simulink library "motor_interface_lib"  (R2022b)
settings: Solver=VariableStepAuto  StartTime=0.0  StopTime=10.0  RelTol=1e-3
undefined symbols (not defined in the file): MI_STATUSES
settings Model: Creator=dr_pa  LastModifiedBy=LinF

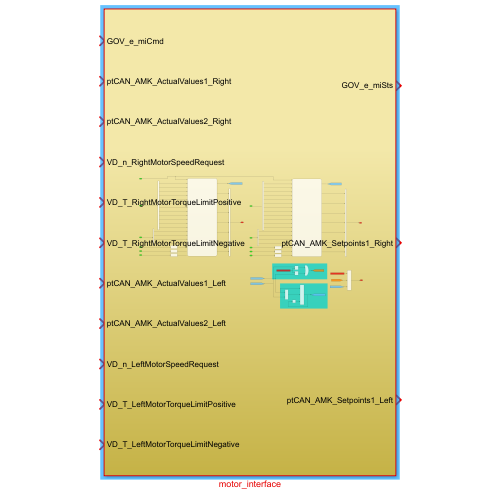
[thumbnail: Simulink's stored preview of the top-level diagram]
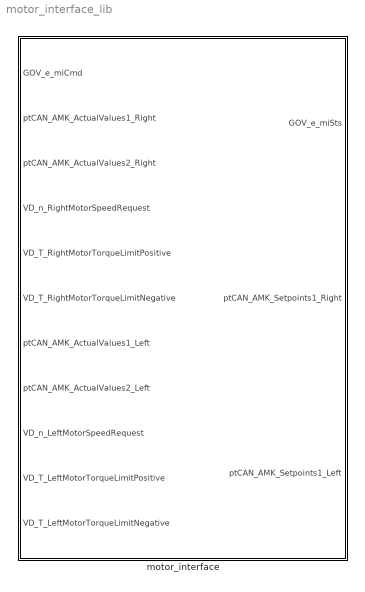
== system motor_interface_lib ==
  motor_interface : Subsystem

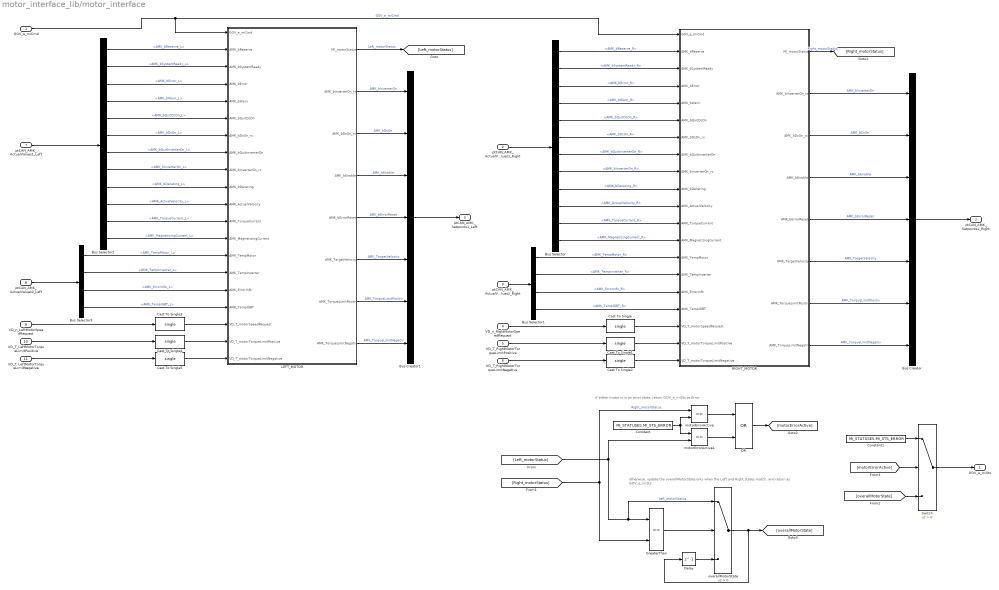
== system motor_interface_lib/motor_interface ==
  note: otherwise, update the overallMotorState only when the Left and Right states match, and return as GOV_e_miSts
  note: if either motor is in an error state, return GOV_e_miSts as Error
  GOV_e_miCmd : Inport
  ptCAN_AMK_ActualValues1_Right : Inport  Port=2
  ptCAN_AMK_ActualValues2_Right : Inport  Port=3
  VD_n_RightMotorSpeedRequest : Inport  Port=4
  VD_T_RightMotorTorqueLimitPositive : Inport  Port=5
  VD_T_RightMotorTorqueLimitNegative : Inport  Port=6
  ptCAN_AMK_ActualValues1_Left : Inport  Port=7
  ptCAN_AMK_ActualValues2_Left : Inport  Port=8
  VD_n_LeftMotorSpeedRequest : Inport  Port=9
  VD_T_LeftMotorTorqueLimitPositive : Inport  Port=10
  VD_T_LeftMotorTorqueLimitNegative : Inport  Port=11
  Bus Creator : BusCreator  Inputs=7
  Bus Creator1 : BusCreator  Inputs=7
  Bus Selector : BusSelector  OutputSignals=AMK_bReserve_R,AMK_bSystemReady_R,AMK_bError_R,AMK_bWarn_R,AMK_bQuitDcOn_R,AMK_bDcOn_R,AMK_bQuitInverterOn_R,AMK_bInverterOn_R,AMK_bDerating_R,AMK_ActualVelocity_R,AMK_TorqueCurrent_R,AMK_MagnetizingCurrent_R
  Bus Selector1 : BusSelector  OutputSignals=AMK_TempMotor_R,AMK_TempInverter_R,AMK_ErrorInfo_R,AMK_TempIGBT_R
  Bus Selector2 : BusSelector  OutputSignals=AMK_bReserve_L,AMK_bSystemReady_L,AMK_bError_L,AMK_bWarn_L,AMK_bQuitDcOn_L,AMK_bDcOn_L,AMK_bQuitInverterOn_L,AMK_bInverterOn_L,AMK_bDerating_L,AMK_ActualVelocity_L,AMK_TorqueCurrent_L,AMK_MagnetizingCurrent_L
  Bus Selector3 : BusSelector  OutputSignals=AMK_TempMotor_L,AMK_TempInverter_L,AMK_ErrorInfo_L,AMK_TempIGBT_L
  Cast To Single{,1..5} (6 alike) : DataTypeConversion  OutDataTypeStr=single  SaturateOnIntegerOverflow=off  RndMeth=Floor
  Constant : Constant  Value=MI_STATUSES.MI_STS_ERROR  OutDataTypeStr=Enum: MI_STATUSES
  Constant1 : Constant  Value=MI_STATUSES.MI_STS_ERROR  OutDataTypeStr=Enum: MI_STATUSES
  Delay : Delay  DelayLength=1  InitialCondition=MI_STATUSES.OFF
  GreaterThan : RelationalOperator  Operator===  OutDataTypeStr=boolean  RndMeth=Simplest  InputSameDT=off
  LEFT_MOTOR : Stateflow chart  TreatAsAtomicUnit=on
  OR : Logic  Operator=OR  IconShape=distinctive  AllPortsSameDT=off  OutDataTypeStr=boolean
  RIGHT_MOTOR : Stateflow chart  TreatAsAtomicUnit=on
  Switch : Switch  Criteria=u2 > Threshold  SaturateOnIntegerOverflow=off  InputSameDT=off
  motorErrorActive : RelationalOperator  Operator===  OutDataTypeStr=boolean  RndMeth=Simplest  InputSameDT=off
  motorErrorActive1 : RelationalOperator  Operator===  OutDataTypeStr=boolean  RndMeth=Simplest  InputSameDT=off
  overallMotorState : Switch  Criteria=u2 > Threshold  SaturateOnIntegerOverflow=off  InputSameDT=off
  GOV_e_miSts : Outport
  ptCAN_AMK_Setpoints1_Right : Outport  Port=2
  ptCAN_AMK_Setpoints1_Left : Outport  Port=3
  wires:
  Cast To Single5/1 -> LEFT_MOTOR/20(VD_T_motorTorqueLimitNegative)
  Cast To Single4/1 -> LEFT_MOTOR/19(VD_T_motorTorqueLimitPositive)
  Cast To Single3/1 -> LEFT_MOTOR/18(VD_T_motorSpeedRequest)
  Cast To Single2/1 -> RIGHT_MOTOR/20(VD_T_motorTorqueLimitNegative)
  Cast To Single1/1 -> RIGHT_MOTOR/19(VD_T_motorTorqueLimitPositive)
  Cast To Single/1 -> RIGHT_MOTOR/18(VD_T_motorSpeedRequest)
  GOV_e_miCmd/1 -> LEFT_MOTOR/1(GOV_e_miCmd), RIGHT_MOTOR/1(GOV_e_miCmd)  "GOV_e_miCmd"
  ptCAN_AMK_ActualValues1_Right/1 -> Bus Selector/1
  Bus Selector/2 -> RIGHT_MOTOR/3(AMK_bSystemReady)  "<AMK_bSystemReady_R>"
  Bus Selector/3 -> RIGHT_MOTOR/4(AMK_bError)  "<AMK_bError_R>"
  Bus Selector/4 -> RIGHT_MOTOR/5(AMK_bWarn)  "<AMK_bWarn_R>"
  Bus Selector/5 -> RIGHT_MOTOR/6(AMK_bQuitDcOn)  "<AMK_bQuitDcOn_R>"
  Bus Selector/6 -> RIGHT_MOTOR/7(AMK_bDcOn_rx)  "<AMK_bDcOn_R>"
  Bus Selector/7 -> RIGHT_MOTOR/8(AMK_bQuitInverterOn)  "<AMK_bQuitInverterOn_R>"
  Bus Selector/8 -> RIGHT_MOTOR/9(AMK_bInverterOn_rx)  "<AMK_bInverterOn_R>"
  Bus Selector/9 -> RIGHT_MOTOR/10(AMK_bDerating)  "<AMK_bDerating_R>"
  Bus Selector/10 -> RIGHT_MOTOR/11(AMK_ActualVelocity)  "<AMK_ActualVelocity_R>"
  Bus Selector/11 -> RIGHT_MOTOR/12(AMK_TorqueCurrent)  "<AMK_TorqueCurrent_R>"
  Bus Selector/12 -> RIGHT_MOTOR/13(AMK_MagnetizingCurrent)  "<AMK_MagnetizingCurrent_R>"
  Bus Selector/1 -> RIGHT_MOTOR/2(AMK_bReserve)  "<AMK_bReserve_R>"
  ptCAN_AMK_ActualValues2_Right/1 -> Bus Selector1/1
  Bus Selector1/1 -> RIGHT_MOTOR/14(AMK_TempMotor)  "<AMK_TempMotor_R>"
  Bus Selector1/2 -> RIGHT_MOTOR/15(AMK_TempInverter)  "<AMK_TempInverter_R>"
  Bus Selector1/3 -> RIGHT_MOTOR/16(AMK_ErrorInfo)  "<AMK_ErrorInfo_R>"
  Bus Selector1/4 -> RIGHT_MOTOR/17(AMK_TempIGBT)  "<AMK_TempIGBT_R>"
  Bus Creator/1 -> ptCAN_AMK_Setpoints1_Right/1
  RIGHT_MOTOR/2(AMK_bInverterOn_tx) -> Bus Creator/1  "AMK_bInverterOn"
  RIGHT_MOTOR/4(AMK_bEnable) -> Bus Creator/3  "AMK_bEnable"
  RIGHT_MOTOR/6(AMK_TargetVelocity) -> Bus Creator/5  "AMK_TargetVelocity"
  RIGHT_MOTOR/3(AMK_bDcOn_tx) -> Bus Creator/2  "AMK_bDcOn"
  RIGHT_MOTOR/5(AMK_bErrorReset) -> Bus Creator/4  "AMK_bErrorReset"
  LEFT_MOTOR/1(MI_motorStatus) -> [Left_motorStatus]  "Left_motorStatus"
  RIGHT_MOTOR/1(MI_motorStatus) -> [Right_motorStatus]  "Right_motorStatus"
  [Left_motorStatus] -> motorErrorActive1/2, overallMotorState/1, GreaterThan/1  "Left_motorStatus"
  [Right_motorStatus] -> motorErrorActive/1, GreaterThan/2  "Right_motorStatus"
  Constant/1 -> motorErrorActive/2, motorErrorActive1/1
  Switch/1 -> GOV_e_miSts/1
  [motorErrorActive] -> Switch/2
  overallMotorState/1 -> Delay/1, [overallMotorState]
  Delay/1 -> overallMotorState/3
  GreaterThan/1 -> overallMotorState/2
  [overallMotorState] -> Switch/3
  OR/1 -> [motorErrorActive]
  motorErrorActive1/1 -> OR/2
  motorErrorActive/1 -> OR/1
  Constant1/1 -> Switch/1
  RIGHT_MOTOR/7(AMK_TorqueLimitPositiv) -> Bus Creator/6  "AMK_TorqueLimitPositiv"
  RIGHT_MOTOR/8(AMK_TorqueLimitNegativ) -> Bus Creator/7  "AMK_TorqueLimitNegativ"
  VD_T_RightMotorTorqueLimitPositive/1 -> Cast To Single1/1
  VD_T_RightMotorTorqueLimitNegative/1 -> Cast To Single2/1
  VD_n_RightMotorSpeedRequest/1 -> Cast To Single/1
  VD_n_LeftMotorSpeedRequest/1 -> Cast To Single3/1
  VD_T_LeftMotorTorqueLimitNegative/1 -> Cast To Single5/1
  VD_T_LeftMotorTorqueLimitPositive/1 -> Cast To Single4/1
  Bus Selector3/4 -> LEFT_MOTOR/17(AMK_TempIGBT)  "<AMK_TempIGBT_L>"
  Bus Selector3/3 -> LEFT_MOTOR/16(AMK_ErrorInfo)  "<AMK_ErrorInfo_L>"
  Bus Selector3/2 -> LEFT_MOTOR/15(AMK_TempInverter)  "<AMK_TempInverter_L>"
  Bus Selector3/1 -> LEFT_MOTOR/14(AMK_TempMotor)  "<AMK_TempMotor_L>"
  Bus Selector2/1 -> LEFT_MOTOR/2(AMK_bReserve)  "<AMK_bReserve_L>"
  Bus Selector2/12 -> LEFT_MOTOR/13(AMK_MagnetizingCurrent)  "<AMK_MagnetizingCurrent_L>"
  Bus Selector2/11 -> LEFT_MOTOR/12(AMK_TorqueCurrent)  "<AMK_TorqueCurrent_L>"
  Bus Selector2/10 -> LEFT_MOTOR/11(AMK_ActualVelocity)  "<AMK_ActualVelocity_L>"
  Bus Selector2/9 -> LEFT_MOTOR/10(AMK_bDerating)  "<AMK_bDerating_L>"
  Bus Selector2/8 -> LEFT_MOTOR/9(AMK_bInverterOn_rx)  "<AMK_bInverterOn_L>"
  Bus Selector2/7 -> LEFT_MOTOR/8(AMK_bQuitInverterOn)  "<AMK_bQuitInverterOn_L>"
  Bus Selector2/6 -> LEFT_MOTOR/7(AMK_bDcOn_rx)  "<AMK_bDcOn_L>"
  Bus Selector2/5 -> LEFT_MOTOR/6(AMK_bQuitDcOn)  "<AMK_bQuitDcOn_L>"
  Bus Selector2/4 -> LEFT_MOTOR/5(AMK_bWarn)  "<AMK_bWarn_L>"
  Bus Selector2/3 -> LEFT_MOTOR/4(AMK_bError)  "<AMK_bError_L>"
  Bus Selector2/2 -> LEFT_MOTOR/3(AMK_bSystemReady)  "<AMK_bSystemReady_L>"
  ptCAN_AMK_ActualValues1_Left/1 -> Bus Selector2/1
  LEFT_MOTOR/8(AMK_TorqueLimitNegativ) -> Bus Creator1/7  "AMK_TorqueLimitNegativ"
  LEFT_MOTOR/7(AMK_TorqueLimitPositiv) -> Bus Creator1/6  "AMK_TorqueLimitPositiv"
  LEFT_MOTOR/5(AMK_bErrorReset) -> Bus Creator1/4  "AMK_bErrorReset"
  LEFT_MOTOR/3(AMK_bDcOn_tx) -> Bus Creator1/2  "AMK_bDcOn"
  LEFT_MOTOR/6(AMK_TargetVelocity) -> Bus Creator1/5  "AMK_TargetVelocity"
  LEFT_MOTOR/4(AMK_bEnable) -> Bus Creator1/3  "AMK_bEnable"
  LEFT_MOTOR/2(AMK_bInverterOn_tx) -> Bus Creator1/1  "AMK_bInverterOn"
  Bus Creator1/1 -> ptCAN_AMK_Setpoints1_Left/1
  ptCAN_AMK_ActualValues2_Left/1 -> Bus Selector3/1

== stateflow chart motor_interface_lib/motor_interface/LEFT_MOTOR ==
  note: [AMK_bError==1]
  state motorOff_waitingForGov
    en:
    MI_motorStatus = MI_STATUSES.OFF;
    AMK_bInverterOn_tx = 0;
    AMK_bDcOn_tx = 0;
    AMK_bEnable = 0;
    AMK_bErrorReset = 0;
    AMK_TargetVelocity = 0;
    AMK_TorqueLimitPositiv = 0;
    AMK_TorqueLimitNegativ = 0;
  state AMK_startup
    state waiting_sysReady
      en:
      MI_motorStatus = MI_STATUSES.STARTUP;
    state toggleDCon
      en:
      AMK_bDcOn_tx = 1;
    state enforceSetpointsZero
      en:
      AMK_TargetVelocity = 0;
      AMK_TorqueLimitPositiv = 0;
      AMK_TorqueLimitNegativ = 0;
    state commandOn
      en:
      AMK_bEnable = 1;
      AMK_bInverterOn_tx = 1;
    waiting_sysReady -> (junction 67) [order 2] : [AMK_bError==1]
    waiting_sysReady -> AMK_startup.toggleDCon [order 1] : [AMK_bSystemReady==1]
    AMK_startup.toggleDCon -> (junction 67) [order 2] : [AMK_bError==1]
    AMK_startup.toggleDCon -> AMK_startup.enforceSetpointsZero [order 1] : [(AMK_bDcOn_rx==1) ...
        | && (AMK_bQuitDcOn==1)]
    AMK_startup.enforceSetpointsZero -> (junction 67) [order 2] : [AMK_bError==1]
    commandOn -> (junction 67) [order 2] : [AMK_bError==1]
    AMK_startup.enforceSetpointsZero -> commandOn [order 1] : after(100,msec)
  state AMK_errorReset
    state toggleReset
      en:
      AMK_bErrorReset = 0;
    state sendReset
      en:
      AMK_bErrorReset = 1;
    state toggleEnable
      en:
      AMK_bEnable = 0;
    state enforceSetpointsZero
      en:
      AMK_TargetVelocity = 0;
      AMK_TorqueLimitPositiv = 0;
      AMK_TorqueLimitNegativ = 0;
      AMK_bInverterOn_tx = 0;
    sendReset -> toggleReset : after(500,msec)
    toggleEnable -> sendReset : after(500,msec)
    AMK_errorReset.enforceSetpointsZero -> toggleEnable : [AMK_bInverterOn_rx==0]
  state AMK_shutdown
    state toggleDCon
      en:
      AMK_bDcOn_tx = 0;
    state commandOff
      en:
      AMK_bEnable = 0;
    state enforceSetpointsZero
      en:
      MI_motorStatus = MI_STATUSES.SHUTDOWN;
      AMK_TargetVelocity = 0;
      AMK_TorqueLimitPositiv = 0;
      AMK_TorqueLimitNegativ = 0;
      AMK_bInverterOn_tx = 0;
    AMK_shutdown.toggleDCon -> (junction 94) [order 2] : [AMK_bError==1]
    commandOff -> AMK_shutdown.toggleDCon [order 1] : [AMK_bQuitInverterOn==0]
    commandOff -> (junction 94) [order 2] : [AMK_bError==1]
    AMK_shutdown.enforceSetpointsZero -> (junction 94) [order 2] : [AMK_bError==1]
    AMK_shutdown.enforceSetpointsZero -> commandOff [order 1] : [AMK_bInverterOn_rx==0]
  state AMK_errorDetected
    en:
    MI_motorStatus = MI_STATUSES.MI_STS_ERROR;
  state AMK_running
    during:
    MI_motorStatus = MI_STATUSES.RUNNING;
    AMK_TargetVelocity = VD_T_motorSpeedRequest;
    AMK_TorqueLimitPositiv = VD_T_motorTorqueLimitPositive;
    AMK_TorqueLimitNegativ = VD_T_motorTorqueLimitNegative;
  toggleReset -> motorOff_waitingForGov : [AMK_bSystemReady==1]
  AMK_running -> AMK_shutdown.enforceSetpointsZero [order 2] : [GOV_e_miCmd == MI_CMD.CMD_SHUTDOWN]
  commandOn -> AMK_running [order 1] : [(AMK_bInverterOn_rx ==1) && ...
      |  (AMK_bQuitInverterOn==1)]
  AMK_shutdown.toggleDCon -> motorOff_waitingForGov [order 1] : [(AMK_bDcOn_rx==0) && (AMK_bQuitDcOn==0)]
  motorOff_waitingForGov -> waiting_sysReady : [GOV_e_miCmd == MI_CMD.CMD_STARTUP]
  (default) -> motorOff_waitingForGov
  (junction 67) -> AMK_errorDetected
  (junction 94) -> AMK_errorDetected
  AMK_errorDetected -> AMK_errorReset.enforceSetpointsZero : [GOV_e_miCmd == MI_CMD.ERR_RESET]
  AMK_running -> AMK_errorDetected [order 1] : [AMK_bError==1]
  data: GOV_e_miCmd input Enum: MI_CMD; MI_motorStatus output Enum: MI_STATUSES size=1; AMK_bReserve input; AMK_bSystemReady input; AMK_bError input; AMK_bWarn input; AMK_bQuitDcOn input; AMK_bDcOn_rx input; AMK_bQuitInverterOn input; AMK_bInverterOn_rx input; AMK_bDerating input; AMK_ActualVelocity input; AMK_TorqueCurrent input; AMK_MagnetizingCurrent input; AMK_TempMotor input; AMK_TempInverter input; AMK_ErrorInfo input; AMK_TempIGBT input; VD_T_motorSpeedRequest input; AMK_bInverterOn_tx output uint8 size=1; AMK_bDcOn_tx output uint8 size=1; AMK_bEnable output uint8 size=1; AMK_bErrorReset output uint8 size=1; AMK_TargetVelocity output single size=1; AMK_TorqueLimitPositiv output single size=1; AMK_TorqueLimitNegativ output single size=1; VD_T_motorTorqueLimitPositive input; VD_T_motorTorqueLimitNegative input

== stateflow chart motor_interface_lib/motor_interface/RIGHT_MOTOR ==
  note: [AMK_bError==1]
  state motorOff_waitingForGov
    en:
    MI_motorStatus = MI_STATUSES.OFF;
    AMK_bInverterOn_tx = 0;
    AMK_bDcOn_tx = 0;
    AMK_bEnable = 0;
    AMK_bErrorReset = 0;
    AMK_TargetVelocity = 0;
    AMK_TorqueLimitPositiv = 0;
    AMK_TorqueLimitNegativ = 0;
  state AMK_startup
    state waiting_sysReady
      en:
      MI_motorStatus = MI_STATUSES.STARTUP;
    state toggleDCon
      en:
      AMK_bDcOn_tx = 1;
    state enforceSetpointsZero
      en:
      AMK_TargetVelocity = 0;
      AMK_TorqueLimitPositiv = 0;
      AMK_TorqueLimitNegativ = 0;
    state commandOn
      en:
      AMK_bEnable = 1;
      AMK_bInverterOn_tx = 1;
    waiting_sysReady -> (junction 67) [order 2] : [AMK_bError==1]
    waiting_sysReady -> AMK_startup.toggleDCon [order 1] : [AMK_bSystemReady==1]
    AMK_startup.toggleDCon -> (junction 67) [order 2] : [AMK_bError==1]
    AMK_startup.toggleDCon -> AMK_startup.enforceSetpointsZero [order 1] : [(AMK_bDcOn_rx==1) ...
        | && (AMK_bQuitDcOn==1)]
    AMK_startup.enforceSetpointsZero -> (junction 67) [order 2] : [AMK_bError==1]
    commandOn -> (junction 67) [order 2] : [AMK_bError==1]
    AMK_startup.enforceSetpointsZero -> commandOn [order 1] : after(100,msec)
  state AMK_errorReset
    state toggleReset
      en:
      AMK_bErrorReset = 0;
    state sendReset
      en:
      AMK_bErrorReset = 1;
    state toggleEnable
      en:
      AMK_bEnable = 0;
    state enforceSetpointsZero
      en:
      AMK_TargetVelocity = 0;
      AMK_TorqueLimitPositiv = 0;
      AMK_TorqueLimitNegativ = 0;
      AMK_bInverterOn_tx = 0;
    sendReset -> toggleReset : after(500,msec)
    toggleEnable -> sendReset : after(500,msec)
    AMK_errorReset.enforceSetpointsZero -> toggleEnable : [AMK_bInverterOn_rx==0]
  state AMK_shutdown
    state toggleDCon
      en:
      AMK_bDcOn_tx = 0;
    state commandOff
      en:
      AMK_bEnable = 0;
    state enforceSetpointsZero
      en:
      MI_motorStatus = MI_STATUSES.SHUTDOWN;
      AMK_TargetVelocity = 0;
      AMK_TorqueLimitPositiv = 0;
      AMK_TorqueLimitNegativ = 0;
      AMK_bInverterOn_tx = 0;
    AMK_shutdown.toggleDCon -> (junction 94) [order 2] : [AMK_bError==1]
    commandOff -> AMK_shutdown.toggleDCon [order 1] : [AMK_bQuitInverterOn==0]
    commandOff -> (junction 94) [order 2] : [AMK_bError==1]
    AMK_shutdown.enforceSetpointsZero -> (junction 94) [order 2] : [AMK_bError==1]
    AMK_shutdown.enforceSetpointsZero -> commandOff [order 1] : [AMK_bInverterOn_rx==0]
  state AMK_errorDetected
    en:
    MI_motorStatus = MI_STATUSES.MI_STS_ERROR;
  state AMK_running
    during:
    MI_motorStatus = MI_STATUSES.RUNNING;
    AMK_TargetVelocity = VD_T_motorSpeedRequest;
    AMK_TorqueLimitPositiv = VD_T_motorTorqueLimitPositive;
    AMK_TorqueLimitNegativ = VD_T_motorTorqueLimitNegative;
  toggleReset -> motorOff_waitingForGov : [AMK_bSystemReady==1]
  AMK_running -> AMK_shutdown.enforceSetpointsZero [order 2] : [GOV_e_miCmd == MI_CMD.CMD_SHUTDOWN]
  commandOn -> AMK_running [order 1] : [(AMK_bInverterOn_rx ==1) && ...
      |  (AMK_bQuitInverterOn==1)]
  AMK_shutdown.toggleDCon -> motorOff_waitingForGov [order 1] : [(AMK_bDcOn_rx==0) && (AMK_bQuitDcOn==0)]
  motorOff_waitingForGov -> waiting_sysReady : [GOV_e_miCmd == MI_CMD.CMD_STARTUP]
  (default) -> motorOff_waitingForGov
  (junction 67) -> AMK_errorDetected
  (junction 94) -> AMK_errorDetected
  AMK_errorDetected -> AMK_errorReset.enforceSetpointsZero : [GOV_e_miCmd == MI_CMD.ERR_RESET]
  AMK_running -> AMK_errorDetected [order 1] : [AMK_bError==1]
  data: GOV_e_miCmd input Enum: MI_CMD; MI_motorStatus output Enum: MI_STATUSES size=1; AMK_bReserve input; AMK_bSystemReady input; AMK_bError input; AMK_bWarn input; AMK_bQuitDcOn input; AMK_bDcOn_rx input; AMK_bQuitInverterOn input; AMK_bInverterOn_rx input; AMK_bDerating input; AMK_ActualVelocity input; AMK_TorqueCurrent input; AMK_MagnetizingCurrent input; AMK_TempMotor input; AMK_TempInverter input; AMK_ErrorInfo input; AMK_TempIGBT input; VD_T_motorSpeedRequest input; AMK_bInverterOn_tx output uint8 size=1; AMK_bDcOn_tx output uint8 size=1; AMK_bEnable output uint8 size=1; AMK_bErrorReset output uint8 size=1; AMK_TargetVelocity output single size=1; AMK_TorqueLimitPositiv output single size=1; AMK_TorqueLimitNegativ output single size=1; VD_T_motorTorqueLimitPositive input; VD_T_motorTorqueLimitNegative input
